simulink model "NPC_PI_SMO"  (R2021b)
settings: Solver=VariableStepAuto  StartTime=0.0  StopTime=3  RelTol=1e-3
values from neighbouring files (symbols this model uses):
  Cdc = 6000e-6    (= 0.006)    [Para_NPC_PI_SMO.m]
  Ki_a = 0.8    [Para_NPC_PI_SMO.m]
  Ki_b = 0    [Para_NPC_PI_SMO.m]
  Ki_c = 40    [Para_NPC_PI_SMO.m]
  Kp_a = 0.09    [Para_NPC_PI_SMO.m]
  Kp_b = 5e-3    (= 0.005)    [Para_NPC_PI_SMO.m]
  Kp_c = 10    [Para_NPC_PI_SMO.m]
  Lline = 2e-3    (= 0.002)    [Para_NPC_PI_SMO.m]
  rho = M + alpha*Cdc*0.3536    (= 10021.216)    [Para_NPC_PI_SMO.m]
  Tc = 1./fc    (= 0.0001)    [Para_NPC_PI_SMO.m]
  Tenable = 0.15    [Para_NPC_PI_SMO.m]
  Tint = 1e-6    (= 1e-06)    [Para_NPC_PI_SMO.m]
  Ts = 1./fs    (= 0.0001)    [Para_NPC_PI_SMO.m]
undefined symbols (not defined in the file or in its folder): DiscIntNeverNeededParam
libraries: spsNeutralLib x12, spsIGBTDiodeLib x12, spsSeriesRLCBranchLib x7, spsDiodeLib x6, slpidlib x4, spsBreakerLib x3, spsVoltageMeasurementLib x3, simulink x2, spsThreePhaseSeriesRLCBranchLib x2, spsabctodq0Lib x2, spsThreePhaseVIMeasurementLib x1, spsThreePhaseBreakerLib x1
settings Model: Creator=Taylor00225  LastModifiedBy=Taylor00225

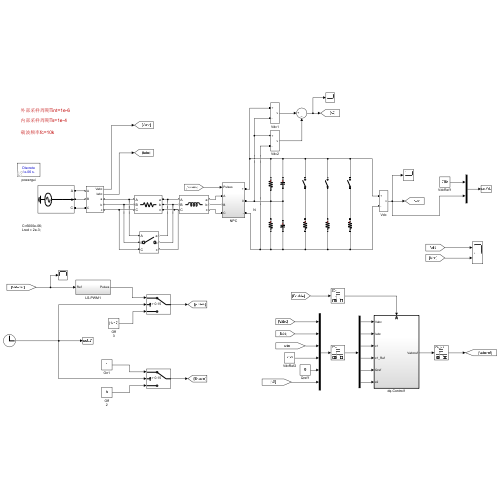
[thumbnail: Simulink's stored preview of the top-level diagram]
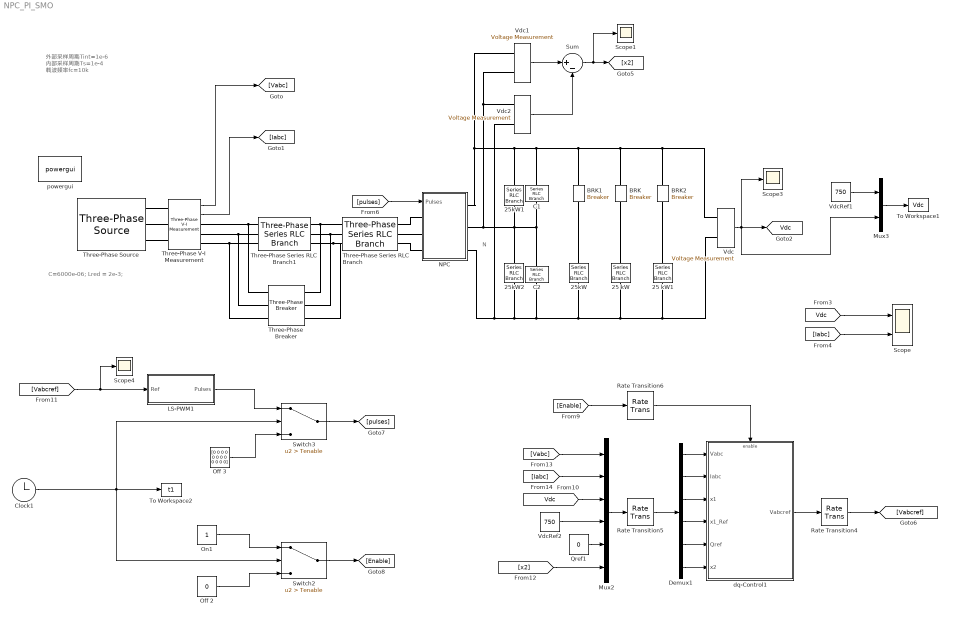
== system NPC_PI_SMO ==
  note: N
  note: 外部采样周期Tint=1e-6
      |
      | 内部采样周期Ts=1e-4
      |
      | 载波频率fc=10k
  note: C=6000e-06;
      | Lred = 2e-3;
  25 kW : spsSeriesRLCBranchLib/Series RLC Branch  LConnTagsString=__new0  RConnTagsString=__new0  BranchType=R  Resistance=360  Inductance=1.0  SetiL0=off  InitialCurrent=0  Capacitance=1.0  Setx0=off  InitialVoltage=0  Measurements=None
  25 kW1 : spsSeriesRLCBranchLib/Series RLC Branch  LConnTagsString=__new0  RConnTagsString=__new0  BranchType=R  Resistance=150  Inductance=1.0  SetiL0=off  InitialCurrent=0  Capacitance=1.0  Setx0=off  InitialVoltage=0  Measurements=None
  25kW : spsSeriesRLCBranchLib/Series RLC Branch  LConnTagsString=__new0  RConnTagsString=__new0  BranchType=R  Resistance=600  Inductance=1.0  SetiL0=off  InitialCurrent=0  Capacitance=1.0  Setx0=off  InitialVoltage=0  Measurements=None
  25kW1 : spsSeriesRLCBranchLib/Series RLC Branch  LConnTagsString=__new0  RConnTagsString=__new0  BranchType=R  Resistance=10e3  Inductance=1.0  SetiL0=off  InitialCurrent=0  Capacitance=1.0  Setx0=off  InitialVoltage=0  Measurements=None
  25kW2 : spsSeriesRLCBranchLib/Series RLC Branch  LConnTagsString=__new0  RConnTagsString=__new0  BranchType=R  Resistance=10e3  Inductance=1.0  SetiL0=off  InitialCurrent=0  Capacitance=1.0  Setx0=off  InitialVoltage=0  Measurements=None
  BRK : spsBreakerLib/Breaker  InitialState=0  SwitchingTimes=[1.2]  External=off  BreakerResistance=0.0001  SnubberResistance=inf  SnubberCapacitance=0  Measurements=None  MoreParameters=off  NoBreakLoop=off
      settings: SourceProductBaseCode=PS
  BRK1 : spsBreakerLib/Breaker  InitialState=0  SwitchingTimes=[0.7]  External=off  BreakerResistance=0.0001  SnubberResistance=inf  SnubberCapacitance=0  Measurements=None  MoreParameters=off  NoBreakLoop=off
      settings: SourceProductBaseCode=PS
  BRK2 : spsBreakerLib/Breaker  InitialState=0  SwitchingTimes=[1.9]  External=off  BreakerResistance=0.0001  SnubberResistance=inf  SnubberCapacitance=0  Measurements=None  MoreParameters=off  NoBreakLoop=off
      settings: SourceProductBaseCode=PS
  C1 : spsSeriesRLCBranchLib/Series RLC Branch  LConnTagsString=__new0  RConnTagsString=__new0  BranchType=C  Resistance=1.0  Inductance=1.0  SetiL0=off  InitialCurrent=0  Capacitance=6000e-06  Setx0=off  InitialVoltage=0  Measurements=None
  C2 : spsSeriesRLCBranchLib/Series RLC Branch  LConnTagsString=__new0  RConnTagsString=__new0  BranchType=C  Resistance=1.0  Inductance=1.0  SetiL0=off  InitialCurrent=0  Capacitance=6000e-06  Setx0=off  InitialVoltage=0  Measurements=None
  Clock1 : Clock
  Demux1 : Demux  Outputs=6
  LS-PWM1 : Subsystem
  Mux2 : Mux  Inputs=6
  Mux3 : Mux  Inputs=2
  NPC : Subsystem
  Off 2 : Constant  Value=0  SampleTime=Tint
  Off 3 : Constant  Value=[0 0 0 0 0 0 0 0 0 0 0 0]  SampleTime=Tint
  On1 : Constant  SampleTime=Tint
  Qref1 : Constant  Value=0  SampleTime=Tint
  Rate Transition4 : RateTransition  Deterministic=off  InitialCondition=[0 0 0]  OutPortSampleTime=Tint
  Rate Transition5 : RateTransition  OutPortSampleTime=Ts
  Rate Transition6 : RateTransition  OutPortSampleTime=Ts
  Scope : Scope  NumInputPorts=2
  Scope1 : Scope
  Scope3 : Scope
  Scope4 : Scope
  Sum : Sum  Inputs=|+-
  Switch2 : Switch  Criteria=u2 > Threshold  Threshold=Tenable
  Switch3 : Switch  Criteria=u2 > Threshold  Threshold=Tenable
  Three-Phase Series RLC Branch : spsThreePhaseSeriesRLCBranchLib/Three-Phase Series RLC Branch  LConnTagsString=A|B|C  RConnTagsString=A|B|C  BranchType=L  Resistance=1  Inductance=Lline  Capacitance=1e-6  Measurements=None
  Three-Phase Series RLC Branch1 : spsThreePhaseSeriesRLCBranchLib/Three-Phase Series RLC Branch  LConnTagsString=A|B|C  RConnTagsString=A|B|C  BranchType=R  Resistance=5  Inductance=2e-3  Capacitance=1e-6  Measurements=None
  Three-Phase V-I Measurement : spsThreePhaseVIMeasurementLib/Three-Phase V-I Measurement  VoltageMeasurement=phase-to-ground  SetLabelV=off  LabelV=Vabc  Vpu=off  VpuLL=off  CurrentMeasurement=yes  SetLabelI=off  LabelI=Iabc  Ipu=off  Pbase=100e6  Vbase=500e3  OutputType=Complex  PhasorSimulation=off  PSBequivalent=0
  Three-Phase Breaker : spsThreePhaseBreakerLib/Three-Phase Breaker  InitialState=open  SwitchA=on  SwitchB=on  SwitchC=on  SwitchTimes=[0.15]  External=off  BreakerResistance=0.00001  SnubberResistance=inf  SnubberCapacitance=0  Measurements=None
  Three-Phase Source : spsThreePhaseSourceLib/Three-Phase Source  InternalConnection=Yg  VoltagePhases=off  Voltage=400  PhaseAngle=0  Voltage_phases=[25e3 25e3 25e3]/sqrt(3)  PhaseAngles_phases=[0 -120 +120]  Frequency=50  NonIdealSource=on  SpecifyImpedance=off  Resistance=0  Inductance=0  ShortCircuitLevel=100e6  BaseVoltage=400  XRratio=7  BusType=swing  Pref=0  Qref=0  Prefabc=[10e3, 10e3, 10e3]  Qrefabc=[0, 0, 0]  Qmin=-inf  Qmax=inf
  To Workspace1 : ToWorkspace  VariableName=Vdc  SampleTime=-1
  To Workspace2 : ToWorkspace  VariableName=t1  SampleTime=-1
  Vdc : spsVoltageMeasurementLib/Voltage Measurement  PhasorSimulation=off  OutputType=Complex  PSBequivalent=0
  Vdc1 : spsVoltageMeasurementLib/Voltage Measurement  PhasorSimulation=off  OutputType=Complex  PSBequivalent=0
  Vdc2 : spsVoltageMeasurementLib/Voltage Measurement  PhasorSimulation=off  OutputType=Complex  PSBequivalent=0
  VdcRef1 : Constant  Value=750  SampleTime=Tint
  VdcRef2 : Constant  Value=750  SampleTime=Tint
  dq-Control1 : Subsystem  TreatAsAtomicUnit=on
  powergui : spspowerguiLib/powergui  Priority=1  SimulationMode=Discrete  SampleTime=Tint  frequency=60  Iterations=50  frequencyindice=0  Pbase=100e6  ErrMax=1e-4  UnitsV=kV  UnitsW=MW  buscounter=0  FunctionMessages=off  echomessages=off  EnableUseOfTLC=off  CurrentSourceSwitches=off  DisableSnubberDevices=off  DisableRonSwitches=off  DisableVfSwitches=off  DisplayEquations=off  AutomaticDiscreteSolvers=off  SolverType=Tustin  Interpol=off  ExternalGateDelay=off  methode=off  Ts=0  x0status=blocks  SPID=off  SwTol=0  HookPort=off  NonlinearTolerance=1e-4  nMaxIteration=100  ContinueOnMaxIteration=off  RestoreLinks=warning  ResistiveCurrentMeasurement=off  Frange=[0:2:500]  Ylog=off  Xlog=on  ShowGrid=off  save=off  variable=ZData  structure=ia  ZoomFFT=off  StartTime=1.9  cycles=5  DisplayStyle=1  fundamental=50  FreqAxis=on  MaxFrequency=2000  frequencyindicesteady=1  RmsSteady=1  display=off
  tag scope: Vdc=global
  wires:
  On1/1 -> Switch2/1
  Rate Transition4/1 -> [Vabcref]
  Off 2/1 -> Switch2/3
  Qref1/1 -> Mux2/5
  Switch3/1 -> [pulses]
  Rate Transition6/1 -> dq-Control1/Enable
  Demux1/6 -> dq-Control1/6(x2)
  Switch2/1 -> [Enable]
  [Enable] -> Rate Transition6/1
  Off 3/1 -> Switch3/3
  LS-PWM1/1(Pulses) -> Switch3/1
  [Vabc] -> Mux2/1
  [Vabcref] -> LS-PWM1/1(Ref), Scope4/1
  Demux1/1 -> dq-Control1/1(Vabc)
  Clock1/1 -> Switch2/2, Switch3/2, To Workspace2/1
  VdcRef2/1 -> Mux2/4
  [Vdc] -> Mux2/3
  Demux1/4 -> dq-Control1/4(x1_Ref)
  dq-Control1/1(Vabcref) -> Rate Transition4/1
  [Iabc] -> Mux2/2
  Mux2/1 -> Rate Transition5/1
  Demux1/2 -> dq-Control1/2(Iabc)
  Demux1/5 -> dq-Control1/5(Qref)
  Rate Transition5/1 -> Demux1/1
  Demux1/3 -> dq-Control1/3(x1)
  [x2] -> Mux2/6
  Sum/1 -> Scope1/1, [x2]
  Vdc2/1 -> Sum/2
  [Iabc] -> Scope/2
  VdcRef1/1 -> Mux3/1
  Three-Phase V-I Measurement/1 -> [Vabc]
  [pulses] -> NPC/1(Pulses)
  Vdc/1 -> Scope3/1, [Vdc], Mux3/2
  Three-Phase V-I Measurement/2 -> [Iabc]
  Vdc1/1 -> Sum/1
  Mux3/1 -> To Workspace1/1
  [Vdc] -> Scope/1
  connections:
  NPC/RConn3 -- Vdc2/LConn2 -- 25 kW/RConn1 -- Vdc/LConn2 -- 25 kW1/RConn1 -- 25kW/RConn1 -- C2/RConn1 -- 25kW2/RConn1
  Three-Phase Breaker/LConn2 -- Three-Phase V-I Measurement/RConn2 -- Three-Phase Series RLC Branch1/LConn2
  Three-Phase Breaker/RConn1 -- Three-Phase Series RLC Branch/LConn1 -- Three-Phase Series RLC Branch1/RConn1
  Three-Phase Breaker/LConn1 -- Three-Phase Series RLC Branch1/LConn1 -- Three-Phase V-I Measurement/RConn1
  Three-Phase Breaker/RConn3 -- Three-Phase Series RLC Branch/LConn3 -- Three-Phase Series RLC Branch1/RConn3
  Three-Phase Breaker/RConn2 -- Three-Phase Series RLC Branch1/RConn2 -- Three-Phase Series RLC Branch/LConn2
  Vdc1/LConn2 -- C1/RConn1 -- C2/LConn1 -- 25kW2/LConn1 -- 25kW1/RConn1 -- NPC/RConn2 -- Vdc2/LConn1
  Three-Phase Breaker/LConn3 -- Three-Phase Series RLC Branch1/LConn3 -- Three-Phase V-I Measurement/RConn3
  BRK/RConn1 -- BRK2/RConn1 -- Vdc/LConn1 -- C1/LConn1 -- 25kW1/LConn1 -- NPC/RConn1 -- Vdc1/LConn1 -- BRK1/RConn1
  BRK1/LConn1 -- 25kW/LConn1
  25 kW1/LConn1 -- BRK2/LConn1
  NPC/LConn1 -- Three-Phase Series RLC Branch/RConn1
  Three-Phase Source/RConn3 -- Three-Phase V-I Measurement/LConn3
  Three-Phase Source/RConn2 -- Three-Phase V-I Measurement/LConn2
  Three-Phase Source/RConn1 -- Three-Phase V-I Measurement/LConn1
  25 kW/LConn1 -- BRK/LConn1
  NPC/LConn2 -- Three-Phase Series RLC Branch/RConn2
  NPC/LConn3 -- Three-Phase Series RLC Branch/RConn3

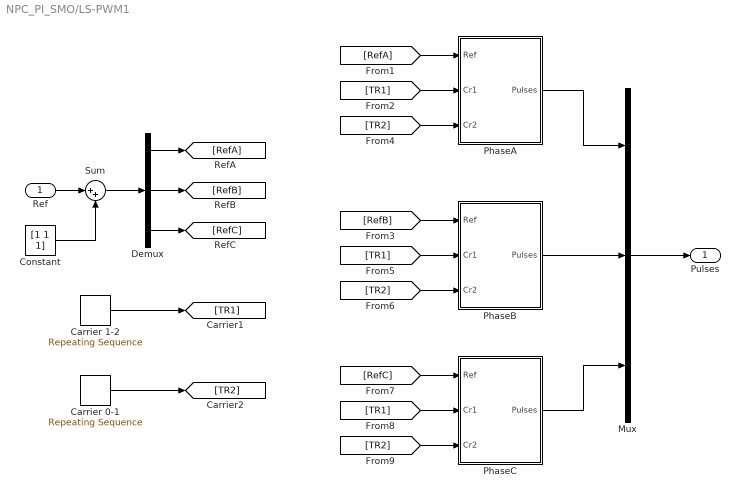
== system NPC_PI_SMO/LS-PWM1 ==
  Ref : Inport
  Carrier 0-1 : simulink/Sources/Repeating Sequence  rep_seq_t=[0 Tc/2 Tc]  rep_seq_y=[0 1 0]
  Carrier 1-2 : simulink/Sources/Repeating Sequence  rep_seq_t=[0 Tc/2 Tc]  rep_seq_y=[1 2 1]
  Constant : Constant  Value=[1 1 1]
  Demux : Demux  Outputs=3
  Mux : Mux  Inputs=3
  PhaseA : Subsystem
  PhaseB : Subsystem
  PhaseC : Subsystem
  Sum : Sum  Inputs=|++
  Pulses : Outport
  wires:
  Mux/1 -> Pulses/1
  PhaseC/1(Pulses) -> Mux/3
  PhaseA/1(Pulses) -> Mux/1
  PhaseB/1(Pulses) -> Mux/2
  [TR2] -> PhaseC/3(Cr2)
  [TR1] -> PhaseC/2(Cr1)
  [RefC] -> PhaseC/1(Ref)
  [TR2] -> PhaseB/3(Cr2)
  [TR1] -> PhaseB/2(Cr1)
  [RefB] -> PhaseB/1(Ref)
  [TR2] -> PhaseA/3(Cr2)
  [TR1] -> PhaseA/2(Cr1)
  [RefA] -> PhaseA/1(Ref)
  Constant/1 -> Sum/2
  Ref/1 -> Sum/1
  Sum/1 -> Demux/1
  Carrier 0-1/1 -> [TR2]
  Carrier 1-2/1 -> [TR1]
  Demux/3 -> [RefC]
  Demux/2 -> [RefB]
  Demux/1 -> [RefA]

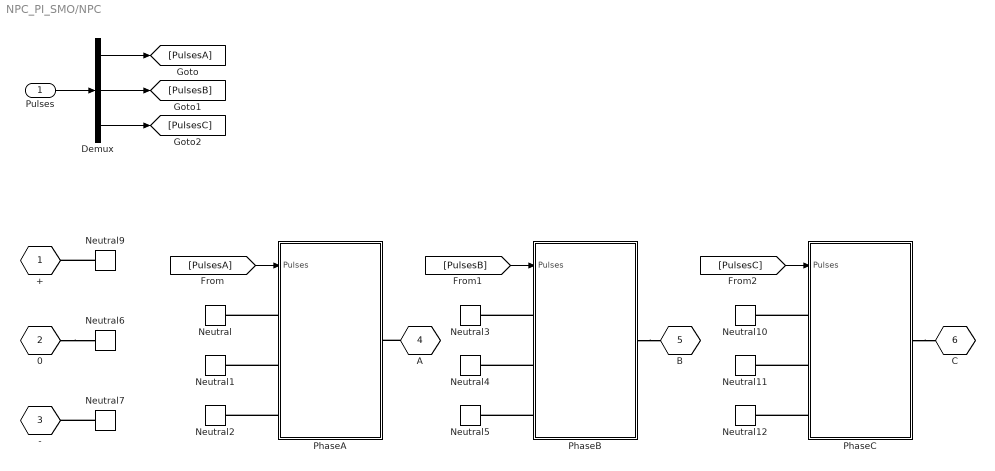
== system NPC_PI_SMO/NPC ==
  Pulses : Inport
  Demux : Demux  Outputs=3
  Neutral{,3,9..10} (4 alike) : spsNeutralLib/Neutral  LConnTagsString=a  NodeNumber=1
      settings: AttributesFormatString=node %<NodeNumber>  SourceProductBaseCode=PS
  Neutral{1,4,6,11} (4 alike) : spsNeutralLib/Neutral  LConnTagsString=a  NodeNumber=2
      settings: AttributesFormatString=node %<NodeNumber>  SourceProductBaseCode=PS
  Neutral{2,5,7,12} (4 alike) : spsNeutralLib/Neutral  LConnTagsString=a  NodeNumber=3
      settings: AttributesFormatString=node %<NodeNumber>  SourceProductBaseCode=PS
  PhaseA : Subsystem
  PhaseB : Subsystem
  PhaseC : Subsystem
  + : PMIOPort  Tag=PMCPort  Side=Right
  0 : PMIOPort  Tag=PMCPort  Port=2  Side=Right
  - : PMIOPort  Tag=PMCPort  Port=3  Side=Right
  A : PMIOPort  Tag=PMCPort  Port=4  Side=Left
  B : PMIOPort  Tag=PMCPort  Port=5  Side=Left
  C : PMIOPort  Tag=PMCPort  Port=6  Side=Left
  wires:
  Pulses/1 -> Demux/1
  Demux/1 -> [PulsesA]
  Demux/2 -> [PulsesB]
  Demux/3 -> [PulsesC]
  [PulsesA] -> PhaseA/1(Pulses)
  [PulsesB] -> PhaseB/1(Pulses)
  [PulsesC] -> PhaseC/1(Pulses)
  connections:
  PhaseA/LConn1 -- Neutral/LConn1
  PhaseA/LConn2 -- Neutral1/LConn1
  PhaseA/LConn3 -- Neutral2/LConn1
  PhaseB/LConn3 -- Neutral5/LConn1
  PhaseB/LConn1 -- Neutral3/LConn1
  PhaseB/LConn2 -- Neutral4/LConn1
  PhaseC/LConn2 -- Neutral11/LConn1
  PhaseC/LConn1 -- Neutral10/LConn1
  PhaseC/LConn3 -- Neutral12/LConn1
  Neutral9/LConn1 -- +/RConn1
  Neutral7/LConn1 -- -/RConn1
  0/RConn1 -- Neutral6/LConn1
  A/RConn1 -- PhaseA/RConn1
  PhaseB/RConn1 -- B/RConn1
  PhaseC/RConn1 -- C/RConn1

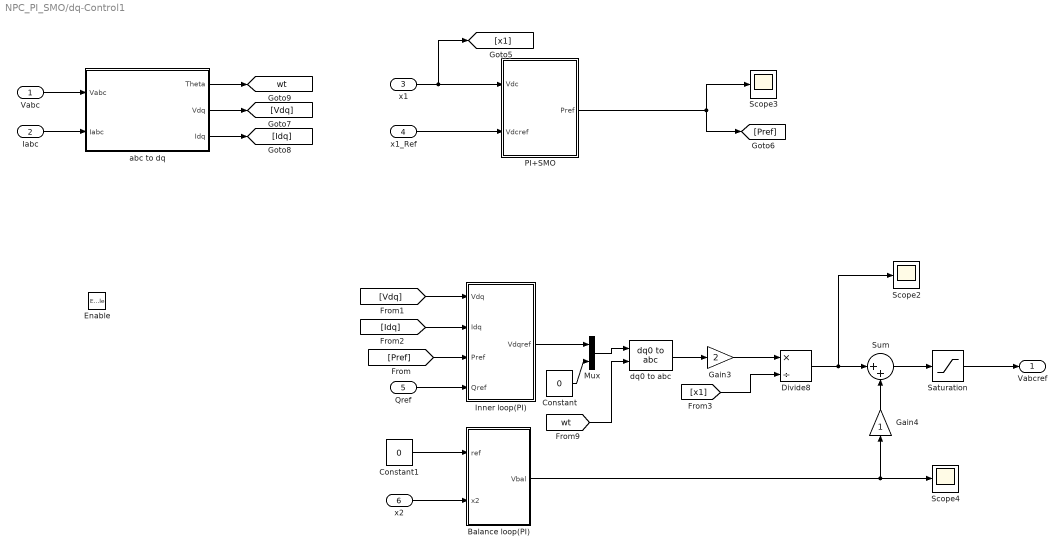
== system NPC_PI_SMO/dq-Control1 ==
  Vabc : Inport  PortDimensions=3
  Iabc : Inport  Port=2  PortDimensions=3
  x1 : Inport  Port=3  PortDimensions=1
  x1_Ref : Inport  Port=4  PortDimensions=1
  Qref : Inport  Port=5  PortDimensions=1
  x2 : Inport  Port=6  PortDimensions=1
  Enable : EnablePort
  Balance loop(PI) : Subsystem
  Constant : Constant  Value=0
  Constant1 : Constant  Value=0
  Divide8 : Product  Inputs=*/
  Gain3 : Gain  Gain=2
  Gain4 : Gain
  Inner loop(PI) : Subsystem
  Mux : Mux  Inputs=[2, 1]
  PI+SMO : Subsystem
  Saturation : Saturate  UpperLimit=1  LowerLimit=-1
  Scope2 : Scope
  Scope3 : Scope
  Scope4 : Scope
  Sum : Sum  Inputs=|++
  abc to dq : Subsystem  TreatAsAtomicUnit=on
  dq0 to abc : spsdq0toabcLib/dq0 to abc  Alignment=Aligned with phase A axis
  Vabcref : Outport  InitialOutput=[0 0 0]
  tag scope: wt=global
  wires:
  x1_Ref/1 -> PI+SMO/2(Vdcref)
  x1/1 -> [x1], PI+SMO/1(Vdc)
  Qref/1 -> Inner loop(PI)/4(Qref)
  [Pref] -> Inner loop(PI)/3(Pref)
  x2/1 -> Balance loop(PI)/2(x2)
  Balance loop(PI)/1(Vbal) -> Scope4/1, Gain4/1
  abc to dq/1(Theta) -> [wt]
  abc to dq/3(Idq) -> [Idq]
  Vabc/1 -> abc to dq/1(Vabc)
  Iabc/1 -> abc to dq/2(Iabc)
  [Vdq] -> Inner loop(PI)/1(Vdq)
  [Idq] -> Inner loop(PI)/2(Idq)
  [wt] -> dq0 to abc/2
  Gain3/1 -> Divide8/1
  Divide8/1 -> Scope2/1, Sum/1
  Sum/1 -> Saturation/1
  dq0 to abc/1 -> Gain3/1
  Saturation/1 -> Vabcref/1
  [x1] -> Divide8/2
  abc to dq/2(Vdq) -> [Vdq]
  Gain4/1 -> Sum/2
  Constant1/1 -> Balance loop(PI)/1(ref)
  PI+SMO/1(Pref) -> [Pref], Scope3/1
  Inner loop(PI)/1(Vdqref) -> Mux/1
  Constant/1 -> Mux/2
  Mux/1 -> dq0 to abc/1

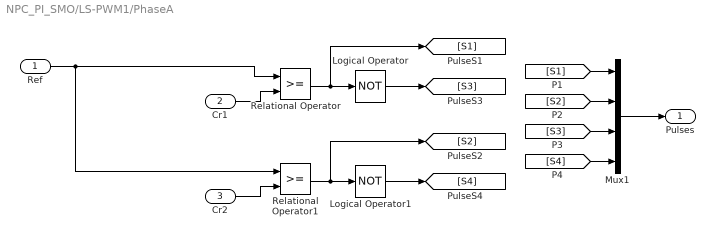
== system NPC_PI_SMO/LS-PWM1/PhaseA ==
  Ref : Inport
  Cr1 : Inport  Port=2
  Cr2 : Inport  Port=3
  Logical Operator : Logic  Operator=NOT  AllPortsSameDT=off  OutDataTypeStr=boolean
  Logical Operator1 : Logic  Operator=NOT  AllPortsSameDT=off  OutDataTypeStr=boolean
  Mux1 : Mux
  Relational Operator : RelationalOperator  OutDataTypeStr=boolean  RndMeth=Nearest
  Relational Operator1 : RelationalOperator  OutDataTypeStr=boolean  RndMeth=Nearest
  Pulses : Outport
  wires:
  Cr1/1 -> Relational Operator/2
  Relational Operator/1 -> Logical Operator/1, [S1]
  Logical Operator/1 -> [S3]
  Ref/1 -> Relational Operator1/1, Relational Operator/1
  Cr2/1 -> Relational Operator1/2
  Relational Operator1/1 -> Logical Operator1/1, [S2]
  Logical Operator1/1 -> [S4]
  Mux1/1 -> Pulses/1
  [S1] -> Mux1/1
  [S2] -> Mux1/2
  [S3] -> Mux1/3
  [S4] -> Mux1/4

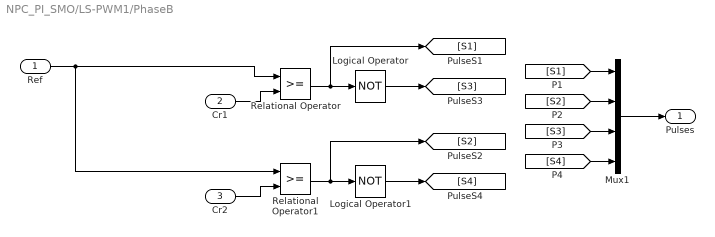
== system NPC_PI_SMO/LS-PWM1/PhaseB ==
  Ref : Inport
  Cr1 : Inport  Port=2
  Cr2 : Inport  Port=3
  Logical Operator : Logic  Operator=NOT  AllPortsSameDT=off  OutDataTypeStr=boolean
  Logical Operator1 : Logic  Operator=NOT  AllPortsSameDT=off  OutDataTypeStr=boolean
  Mux1 : Mux
  Relational Operator : RelationalOperator  OutDataTypeStr=boolean  RndMeth=Nearest
  Relational Operator1 : RelationalOperator  OutDataTypeStr=boolean  RndMeth=Nearest
  Pulses : Outport
  wires:
  [S4] -> Mux1/4
  [S3] -> Mux1/3
  [S2] -> Mux1/2
  [S1] -> Mux1/1
  Mux1/1 -> Pulses/1
  Logical Operator1/1 -> [S4]
  Relational Operator1/1 -> [S2], Logical Operator1/1
  Cr2/1 -> Relational Operator1/2
  Ref/1 -> Relational Operator/1, Relational Operator1/1
  Logical Operator/1 -> [S3]
  Relational Operator/1 -> [S1], Logical Operator/1
  Cr1/1 -> Relational Operator/2

== system NPC_PI_SMO/LS-PWM1/PhaseC ==
  Ref : Inport
  Cr1 : Inport  Port=2
  Cr2 : Inport  Port=3
  Logical Operator : Logic  Operator=NOT  AllPortsSameDT=off  OutDataTypeStr=boolean
  Logical Operator1 : Logic  Operator=NOT  AllPortsSameDT=off  OutDataTypeStr=boolean
  Mux1 : Mux
  Relational Operator : RelationalOperator  OutDataTypeStr=boolean  RndMeth=Nearest
  Relational Operator1 : RelationalOperator  OutDataTypeStr=boolean  RndMeth=Nearest
  Pulses : Outport
  wires:
  Cr1/1 -> Relational Operator/2
  Relational Operator/1 -> Logical Operator/1, [S1]
  Logical Operator/1 -> [S3]
  Ref/1 -> Relational Operator1/1, Relational Operator/1
  Cr2/1 -> Relational Operator1/2
  Relational Operator1/1 -> Logical Operator1/1, [S2]
  Logical Operator1/1 -> [S4]
  Mux1/1 -> Pulses/1
  [S1] -> Mux1/1
  [S2] -> Mux1/2
  [S3] -> Mux1/3
  [S4] -> Mux1/4

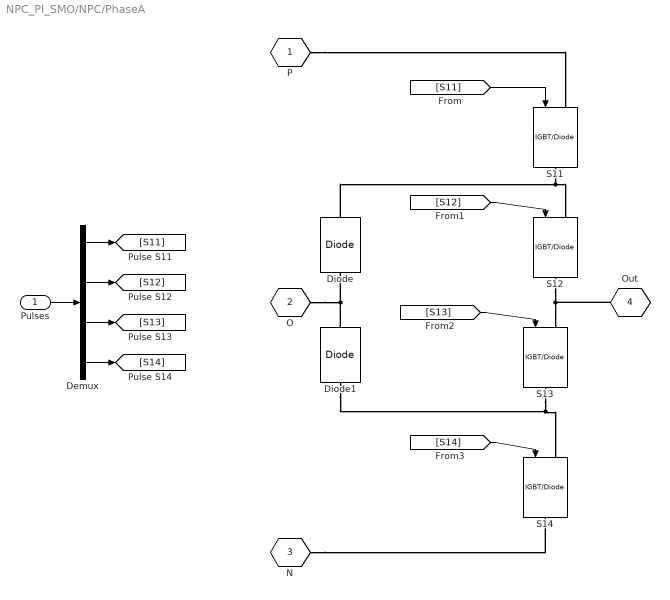
== system NPC_PI_SMO/NPC/PhaseA ==
  Pulses : Inport
  Demux : Demux
  Diode : spsDiodeLib/Diode  Ron=0.001  Lon=0  Vf=0.8  IC=0  UseSnubber=off  Rs=1e5  Cs=inf  Measurements=off
  Diode1 : spsDiodeLib/Diode  Ron=0.001  Lon=0  Vf=0.8  IC=0  UseSnubber=off  Rs=1e5  Cs=inf  Measurements=off
  S{11..14} (4 alike) : spsIGBTDiodeLib/IGBT//Diode  Ron=1e-3  Rs=1e5  Cs=inf  Measurements=off
  P : PMIOPort  Tag=PMCPort  Side=Left
  O : PMIOPort  Tag=PMCPort  Port=2  Side=Left
  N : PMIOPort  Tag=PMCPort  Port=3  Side=Left
  Out : PMIOPort  Tag=PMCPort  Port=4  Side=Right
  wires:
  Pulses/1 -> Demux/1
  Demux/1 -> [S11]
  Demux/3 -> [S13]
  Demux/2 -> [S12]
  Demux/4 -> [S14]
  [S11] -> S11/1
  [S12] -> S12/1
  [S13] -> S13/1
  [S14] -> S14/1
  connections:
  S11/RConn1 -- S12/LConn1 -- Diode/RConn1
  S13/RConn1 -- Diode1/LConn1 -- S14/LConn1
  Diode1/RConn1 -- O/RConn1 -- Diode/LConn1
  S12/RConn1 -- Out/RConn1 -- S13/LConn1
  P/RConn1 -- S11/LConn1
  N/RConn1 -- S14/RConn1

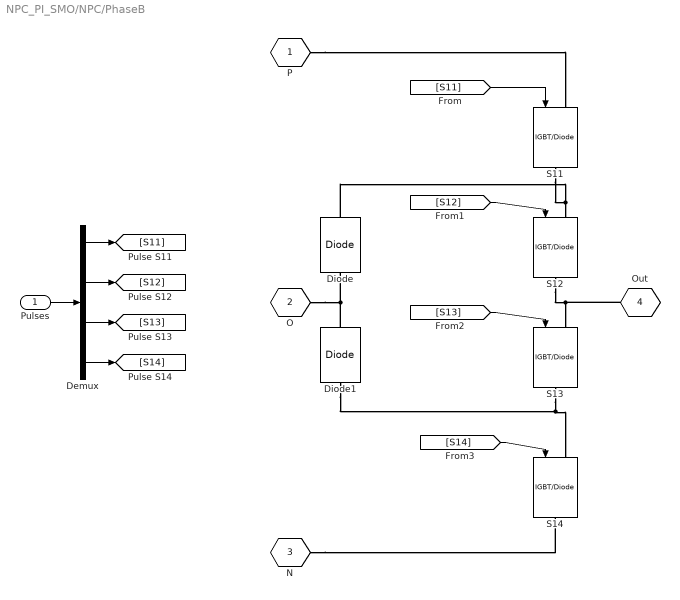
== system NPC_PI_SMO/NPC/PhaseB ==
  Pulses : Inport
  Demux : Demux
  Diode : spsDiodeLib/Diode  Ron=0.001  Lon=0  Vf=0.8  IC=0  UseSnubber=off  Rs=1e5  Cs=inf  Measurements=off
  Diode1 : spsDiodeLib/Diode  Ron=0.001  Lon=0  Vf=0.8  IC=0  UseSnubber=off  Rs=1e5  Cs=inf  Measurements=off
  S{11..14} (4 alike) : spsIGBTDiodeLib/IGBT//Diode  Ron=1e-3  Rs=1e5  Cs=inf  Measurements=off
  P : PMIOPort  Tag=PMCPort  Side=Left
  O : PMIOPort  Tag=PMCPort  Port=2  Side=Left
  N : PMIOPort  Tag=PMCPort  Port=3  Side=Left
  Out : PMIOPort  Tag=PMCPort  Port=4  Side=Right
  wires:
  [S14] -> S14/1
  [S13] -> S13/1
  [S12] -> S12/1
  [S11] -> S11/1
  Demux/4 -> [S14]
  Demux/2 -> [S12]
  Demux/3 -> [S13]
  Demux/1 -> [S11]
  Pulses/1 -> Demux/1
  connections:
  N/RConn1 -- S14/RConn1
  P/RConn1 -- S11/LConn1
  Out/RConn1 -- S13/LConn1 -- S12/RConn1
  O/RConn1 -- Diode1/RConn1 -- Diode/LConn1
  Diode1/LConn1 -- S13/RConn1 -- S14/LConn1
  S12/LConn1 -- S11/RConn1 -- Diode/RConn1

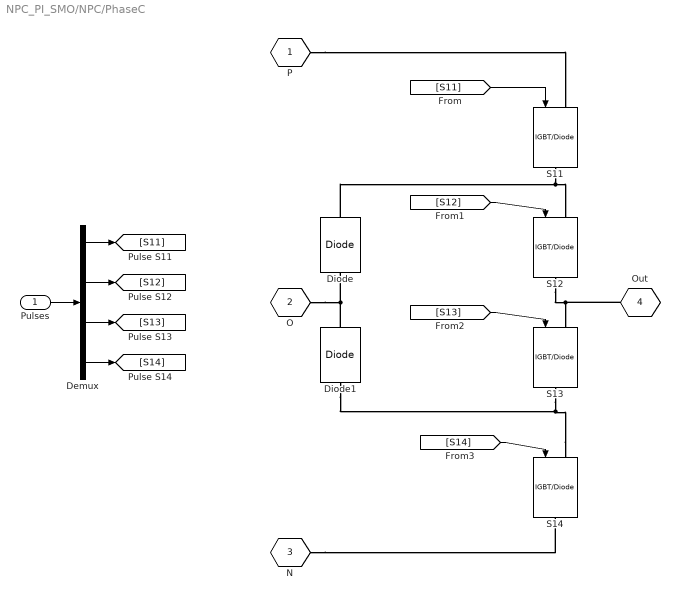
== system NPC_PI_SMO/NPC/PhaseC ==
  Pulses : Inport
  Demux : Demux
  Diode : spsDiodeLib/Diode  Ron=0.001  Lon=0  Vf=0.8  IC=0  UseSnubber=off  Rs=1e5  Cs=inf  Measurements=off
  Diode1 : spsDiodeLib/Diode  Ron=0.001  Lon=0  Vf=0.8  IC=0  UseSnubber=off  Rs=1e5  Cs=inf  Measurements=off
  S{11..14} (4 alike) : spsIGBTDiodeLib/IGBT//Diode  Ron=1e-3  Rs=1e5  Cs=inf  Measurements=off
  P : PMIOPort  Tag=PMCPort  Side=Left
  O : PMIOPort  Tag=PMCPort  Port=2  Side=Left
  N : PMIOPort  Tag=PMCPort  Port=3  Side=Left
  Out : PMIOPort  Tag=PMCPort  Port=4  Side=Right
  wires:
  Pulses/1 -> Demux/1
  Demux/1 -> [S11]
  Demux/3 -> [S13]
  Demux/2 -> [S12]
  Demux/4 -> [S14]
  [S11] -> S11/1
  [S12] -> S12/1
  [S13] -> S13/1
  [S14] -> S14/1
  connections:
  Diode/RConn1 -- S11/RConn1 -- S12/LConn1
  S14/LConn1 -- S13/RConn1 -- Diode1/LConn1
  Diode/LConn1 -- Diode1/RConn1 -- O/RConn1
  S12/RConn1 -- S13/LConn1 -- Out/RConn1
  P/RConn1 -- S11/LConn1
  N/RConn1 -- S14/RConn1

== system NPC_PI_SMO/dq-Control1/Balance loop(PI) ==
  ref : Inport
  x2 : Inport  Port=2
  PID Controller4 : slpidlib/PID Controller  Controller=PID  Form=Parallel  TimeDomain=Discrete-time  UseExternalTs=off  SampleTime=Ts  IntegratorMethod=Forward Euler  FilterMethod=Forward Euler  ControllerParametersSource=internal  P=Kp_b  I=Ki_b  D=0  UseFilter=on  N=0  TunerSelectOption=Transfer Function Based (PID Tuner App)  InitialConditionSource=internal  InitialConditionForIntegrator=0  InitialConditionForFilter=0  DifferentiatorICPrevScaledInput=0  ExternalReset=none  TrackingMode=off  Kt=1  LimitOutput=off  SatLimitsSource=internal  UpperSaturationLimit=inf  LowerSaturationLimit=-inf  LinearizeAsGain=on  AntiWindupMode=none  Kb=1  POutMin=[]  POutMax=[]  IOutMin=[]  IOutMax=[]  DOutMin=[]  DOutMax=[]  NOutMin=[]  NOutMax=[]  SumOutMin=[]  SumOutMax=[]  SaturationOutMin=[]  SaturationOutMax=[]  PParamMin=[]  PParamMax=[]  IParamMin=[]  IParamMax=[]  DParamMin=[]  DParamMax=[]  NParamMin=[]  NParamMax=[]  KbParamMin=[]  KbParamMax=[]  KtParamMin=[]  KtParamMax=[]  KbOutMin=[]  KbOutMax=[]  KtOutMin=[]  KtOutMax=[]  IntegratorOutMin=[]  IntegratorOutMax=[]  FilterOutMin=[]  FilterOutMax=[]  SumI1OutMin=[]  SumI1OutMax=[]  SumI2OutMin=[]  SumI2OutMax=[]  SumI3OutMin=[]  SumI3OutMax=[]  SumI4OutMin=[]  SumI4OutMax=[]  SumDOutMin=[]  SumDOutMax=[]  DifferentiatorOutMin=[]  DifferentiatorOutMax=[]  FilterDiffOutCoefMin=[]  FilterDiffOutCoefMax=[]  ReciprocalOutMin=[]  ReciprocalOutMax=[]  SumDenOutMin=[]  SumDenOutMax=[]  SumNumOutMin=[]  SumNumOutMax=[]  DivideOutMin=[]  DivideOutMax=[]  UdiffTsProdOutMin=[]  UdiffTsProdOutMax=[]  NTsProdOutMin=[]  NTsProdOutMax=[]  UintegralTsProdOutMin=[]  UintegralTsProdOutMax=[]  UngainTsProdOutMin=[]  UngainTsProdOutMax=[]  IntegratorContinuousStateAttributes=''  IntegratorStateMustResolveToSignalObject=off  IntegratorRTWStateStorageClass=Auto  FilterContinuousStateAttributes=''  FilterStateMustResolveToSignalObject=off  FilterRTWStateStorageClass=Auto  ParallelPVariant=InternalParameters  IdealPVariant=Disabled  IVariant=InternalParameters  DVariant=InternalParameters  IntegratorVariant=Discrete  SatVariant=Disabled  AWVariant=Passthrough  PCopyVariant=Disabled  TRVariant=Disabled  FdbkBlocksVariant=Forward  IdealPFdbkVariant=Disabled  SatFdbkVariant=Disabled  DerivativeFilterVariant=ForwardEulerFilter  NVariant=InternalParameters  NCopyVariant=Disabled  FilterICVariant=InternalICsFilter  IntegratorICVariant=InternalICs  ExternalResetVariant=Disabled  TRSumVariant=Passthrough  SumFdbkVariant=Disabled  SumVariant=Sum_PID  TsampFilterVariant=InternalTs  TsampNgainVariant=Passthrough  TsampIntegralVariant=Passthrough  ExternalSaturationOutDataTypeStr=Inherit: Same as second input
  Sum1 : Sum  Inputs=|+-
  Vbal : Outport
  wires:
  PID Controller4/1 -> Vbal/1
  ref/1 -> Sum1/1
  x2/1 -> Sum1/2
  Sum1/1 -> PID Controller4/1

== system NPC_PI_SMO/dq-Control1/Inner loop(PI) ==
  Vdq : Inport
  Idq : Inport  Port=2
  Pref : Inport  Port=3
  Qref : Inport  Port=4
  Demux : Demux  Outputs=2
  Demux1 : Demux  Outputs=2
  Idq Control : Subsystem
  Idqref Calculation : Subsystem
  Mux : Mux  Inputs=2
  Scope3 : Scope
  Vdqref : Outport  InitialOutput=[0 0 0]
  wires:
  Vdq/1 -> Idqref Calculation/1(Vdq)
  Qref/1 -> Idqref Calculation/3(Qref)
  Pref/1 -> Idqref Calculation/2(Pref)
  Idqref Calculation/1(IdqRef) -> [Idqref]
  [Idqref] -> Idq Control/1(Idqref), Demux1/1
  Idq/1 -> Demux/1, Idq Control/2(Idq)
  Idq Control/1(Vdqref) -> Vdqref/1
  Demux1/1 -> Mux/1
  Demux/1 -> Mux/2
  Mux/1 -> Scope3/1

== system NPC_PI_SMO/dq-Control1/PI+SMO ==
  Vdc : Inport
  Vdcref : Inport  Port=2
  Discrete PID Controller : slpidlib/PID Controller  Controller=PI  Form=Parallel  TimeDomain=Discrete-time  UseExternalTs=off  SampleTime=-1  IntegratorMethod=Forward Euler  FilterMethod=Forward Euler  ControllerParametersSource=internal  P=Kp_a  I=Ki_a  D=0  UseFilter=on  N=0  TunerSelectOption=Transfer Function Based (PID Tuner App)  InitialConditionSource=internal  InitialConditionForIntegrator=0  InitialConditionForFilter=0  DifferentiatorICPrevScaledInput=0  ExternalReset=none  TrackingMode=off  Kt=1  LimitOutput=off  SatLimitsSource=internal  UpperSaturationLimit=inf  LowerSaturationLimit=-inf  LinearizeAsGain=off  AntiWindupMode=none  Kb=1  POutMin=[]  POutMax=[]  IOutMin=[]  IOutMax=[]  DOutMin=[]  DOutMax=[]  NOutMin=[]  NOutMax=[]  SumOutMin=[]  SumOutMax=[]  SaturationOutMin=[]  SaturationOutMax=[]  PParamMin=[]  PParamMax=[]  IParamMin=[]  IParamMax=[]  DParamMin=[]  DParamMax=[]  NParamMin=[]  NParamMax=[]  KbParamMin=[]  KbParamMax=[]  KtParamMin=[]  KtParamMax=[]  KbOutMin=[]  KbOutMax=[]  KtOutMin=[]  KtOutMax=[]  IntegratorOutMin=[]  IntegratorOutMax=[]  FilterOutMin=[]  FilterOutMax=[]  SumI1OutMin=[]  SumI1OutMax=[]  SumI2OutMin=[]  SumI2OutMax=[]  SumI3OutMin=[]  SumI3OutMax=[]  SumI4OutMin=[]  SumI4OutMax=[]  SumDOutMin=[]  SumDOutMax=[]  DifferentiatorOutMin=[]  DifferentiatorOutMax=[]  FilterDiffOutCoefMin=[]  FilterDiffOutCoefMax=[]  ReciprocalOutMin=[]  ReciprocalOutMax=[]  SumDenOutMin=[]  SumDenOutMax=[]  SumNumOutMin=[]  SumNumOutMax=[]  DivideOutMin=[]  DivideOutMax=[]  UdiffTsProdOutMin=[]  UdiffTsProdOutMax=[]  NTsProdOutMin=[]  NTsProdOutMax=[]  UintegralTsProdOutMin=[]  UintegralTsProdOutMax=[]  UngainTsProdOutMin=[]  UngainTsProdOutMax=[]  IntegratorContinuousStateAttributes=''  IntegratorStateMustResolveToSignalObject=off  IntegratorRTWStateStorageClass=Auto  FilterContinuousStateAttributes=''  FilterStateMustResolveToSignalObject=off  FilterRTWStateStorageClass=Auto  ParallelPVariant=InternalParameters  IdealPVariant=Disabled  IVariant=InternalParameters  DVariant=Disabled  IntegratorVariant=Discrete  SatVariant=Disabled  AWVariant=Passthrough  PCopyVariant=Disabled  TRVariant=Disabled  FdbkBlocksVariant=Forward  IdealPFdbkVariant=Disabled  SatFdbkVariant=Disabled  DerivativeFilterVariant=Disabled  NVariant=Disabled  NCopyVariant=Disabled_SignalSpec  FilterICVariant=Disabled  IntegratorICVariant=InternalICs  ExternalResetVariant=Disabled  TRSumVariant=Passthrough  SumFdbkVariant=Disabled  SumVariant=Sum_PI  TsampFilterVariant=InternalTs  TsampNgainVariant=Passthrough  TsampIntegralVariant=Passthrough  ExternalSaturationOutDataTypeStr=Inherit: Same as second input
  Gain : Gain  Gain=0.5
  Gain2 : Gain  Gain=0.5
  Product : Product
  Product1 : Product
  SMO : Subsystem
  Sum : Sum  Inputs=|-+
  Sum1 : Sum  Inputs=|++
  Pref : Outport
  wires:
  Discrete PID Controller/1 -> Sum1/1, SMO/1(ud)
  [zref] -> Sum/2
  Gain2/1 -> [zref]
  Product1/1 -> Gain2/1
  Gain/1 -> [z]
  Product/1 -> Gain/1
  Vdcref/1 -> Product1/1, Product1/2
  Vdc/1 -> Product/1, Product/2
  Sum/1 -> Discrete PID Controller/1
  [z] -> SMO/2(y)
  Sum1/1 -> Pref/1
  [z] -> Sum/1
  SMO/1(disturb) -> Sum1/2

== system NPC_PI_SMO/dq-Control1/abc to dq ==
  Vabc : Inport
  Iabc : Inport  Port=2
  Demux : Demux  Outputs=[2, 1]
  Demux1 : Demux  Outputs=[2, 1]
  PLL (3ph) : spsPLL3phLib/PLL (3ph)  Fmin=45  Par_Init=[0, 50]  ParK=[180, 3200, 1]  TcD=1e-4  MaxRateChangeFreq=12  FilterCutOffFreq=25  Ts=Ts  AGC=on
  abc to dq0 : spsabctodq0Lib/abc to dq0  Alignment=Aligned with phase A axis
  abc to dq1 : spsabctodq0Lib/abc to dq0  Alignment=Aligned with phase A axis
  Theta : Outport
  Vdq : Outport  Port=2
  Idq : Outport  Port=3
  wires:
  Vabc/1 -> abc to dq0/1, PLL (3ph)/1
  [Theta] -> Theta/1
  PLL (3ph)/2 -> abc to dq0/2, [Theta]
  Iabc/1 -> abc to dq1/1
  [Theta] -> abc to dq1/2
  abc to dq0/1 -> Demux/1
  Demux/1 -> Vdq/1
  abc to dq1/1 -> Demux1/1
  Demux1/1 -> Idq/1

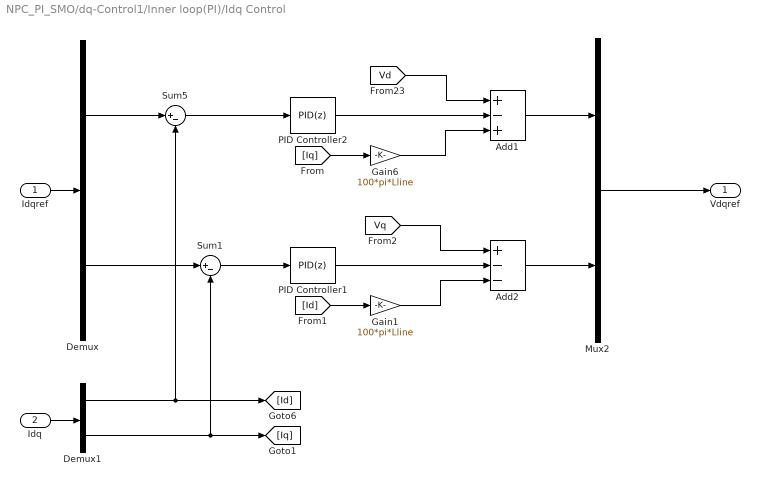
== system NPC_PI_SMO/dq-Control1/Inner loop(PI)/Idq Control ==
  Idqref : Inport
  Idq : Inport  Port=2
  Add1 : Sum  Inputs=+-+
  Add2 : Sum  Inputs=+--
  Demux : Demux  Outputs=2
  Demux1 : Demux  Outputs=2
  Gain1 : Gain  Gain=100*pi*Lline
  Gain6 : Gain  Gain=100*pi*Lline
  Mux2 : Mux  Inputs=2
  PID Controller1 : slpidlib/PID Controller  Controller=PID  Form=Parallel  TimeDomain=Discrete-time  UseExternalTs=off  SampleTime=Ts  IntegratorMethod=Forward Euler  FilterMethod=Forward Euler  ControllerParametersSource=internal  P=Kp_c  I=Ki_c  D=0  UseFilter=on  N=0  TunerSelectOption=Transfer Function Based (PID Tuner App)  InitialConditionSource=internal  InitialConditionForIntegrator=0  InitialConditionForFilter=0  DifferentiatorICPrevScaledInput=0  ExternalReset=none  TrackingMode=off  Kt=1  LimitOutput=off  SatLimitsSource=internal  UpperSaturationLimit=inf  LowerSaturationLimit=-inf  LinearizeAsGain=on  AntiWindupMode=none  Kb=1  POutMin=[]  POutMax=[]  IOutMin=[]  IOutMax=[]  DOutMin=[]  DOutMax=[]  NOutMin=[]  NOutMax=[]  SumOutMin=[]  SumOutMax=[]  SaturationOutMin=[]  SaturationOutMax=[]  PParamMin=[]  PParamMax=[]  IParamMin=[]  IParamMax=[]  DParamMin=[]  DParamMax=[]  NParamMin=[]  NParamMax=[]  KbParamMin=[]  KbParamMax=[]  KtParamMin=[]  KtParamMax=[]  KbOutMin=[]  KbOutMax=[]  KtOutMin=[]  KtOutMax=[]  IntegratorOutMin=[]  IntegratorOutMax=[]  FilterOutMin=[]  FilterOutMax=[]  SumI1OutMin=[]  SumI1OutMax=[]  SumI2OutMin=[]  SumI2OutMax=[]  SumI3OutMin=[]  SumI3OutMax=[]  SumI4OutMin=[]  SumI4OutMax=[]  SumDOutMin=[]  SumDOutMax=[]  DifferentiatorOutMin=[]  DifferentiatorOutMax=[]  FilterDiffOutCoefMin=[]  FilterDiffOutCoefMax=[]  ReciprocalOutMin=[]  ReciprocalOutMax=[]  SumDenOutMin=[]  SumDenOutMax=[]  SumNumOutMin=[]  SumNumOutMax=[]  DivideOutMin=[]  DivideOutMax=[]  UdiffTsProdOutMin=[]  UdiffTsProdOutMax=[]  NTsProdOutMin=[]  NTsProdOutMax=[]  UintegralTsProdOutMin=[]  UintegralTsProdOutMax=[]  UngainTsProdOutMin=[]  UngainTsProdOutMax=[]  IntegratorContinuousStateAttributes=''  IntegratorStateMustResolveToSignalObject=off  IntegratorRTWStateStorageClass=Auto  FilterContinuousStateAttributes=''  FilterStateMustResolveToSignalObject=off  FilterRTWStateStorageClass=Auto  ParallelPVariant=InternalParameters  IdealPVariant=Disabled  IVariant=InternalParameters  DVariant=InternalParameters  IntegratorVariant=Discrete  SatVariant=Disabled  AWVariant=Passthrough  PCopyVariant=Disabled  TRVariant=Disabled  FdbkBlocksVariant=Forward  IdealPFdbkVariant=Disabled  SatFdbkVariant=Disabled  DerivativeFilterVariant=ForwardEulerFilter  NVariant=InternalParameters  NCopyVariant=Disabled  FilterICVariant=InternalICsFilter  IntegratorICVariant=InternalICs  ExternalResetVariant=Disabled  TRSumVariant=Passthrough  SumFdbkVariant=Disabled  SumVariant=Sum_PID  TsampFilterVariant=InternalTs  TsampNgainVariant=Passthrough  TsampIntegralVariant=Passthrough  ExternalSaturationOutDataTypeStr=Inherit: Same as second input
  PID Controller2 : slpidlib/PID Controller  Controller=PID  Form=Parallel  TimeDomain=Discrete-time  UseExternalTs=off  SampleTime=Ts  IntegratorMethod=Forward Euler  FilterMethod=Forward Euler  ControllerParametersSource=internal  P=Kp_c  I=Ki_c  D=0  UseFilter=on  N=0  TunerSelectOption=Transfer Function Based (PID Tuner App)  InitialConditionSource=internal  InitialConditionForIntegrator=0  InitialConditionForFilter=0  DifferentiatorICPrevScaledInput=0  ExternalReset=none  TrackingMode=off  Kt=1  LimitOutput=off  SatLimitsSource=internal  UpperSaturationLimit=inf  LowerSaturationLimit=-inf  LinearizeAsGain=on  AntiWindupMode=none  Kb=1  POutMin=[]  POutMax=[]  IOutMin=[]  IOutMax=[]  DOutMin=[]  DOutMax=[]  NOutMin=[]  NOutMax=[]  SumOutMin=[]  SumOutMax=[]  SaturationOutMin=[]  SaturationOutMax=[]  PParamMin=[]  PParamMax=[]  IParamMin=[]  IParamMax=[]  DParamMin=[]  DParamMax=[]  NParamMin=[]  NParamMax=[]  KbParamMin=[]  KbParamMax=[]  KtParamMin=[]  KtParamMax=[]  KbOutMin=[]  KbOutMax=[]  KtOutMin=[]  KtOutMax=[]  IntegratorOutMin=[]  IntegratorOutMax=[]  FilterOutMin=[]  FilterOutMax=[]  SumI1OutMin=[]  SumI1OutMax=[]  SumI2OutMin=[]  SumI2OutMax=[]  SumI3OutMin=[]  SumI3OutMax=[]  SumI4OutMin=[]  SumI4OutMax=[]  SumDOutMin=[]  SumDOutMax=[]  DifferentiatorOutMin=[]  DifferentiatorOutMax=[]  FilterDiffOutCoefMin=[]  FilterDiffOutCoefMax=[]  ReciprocalOutMin=[]  ReciprocalOutMax=[]  SumDenOutMin=[]  SumDenOutMax=[]  SumNumOutMin=[]  SumNumOutMax=[]  DivideOutMin=[]  DivideOutMax=[]  UdiffTsProdOutMin=[]  UdiffTsProdOutMax=[]  NTsProdOutMin=[]  NTsProdOutMax=[]  UintegralTsProdOutMin=[]  UintegralTsProdOutMax=[]  UngainTsProdOutMin=[]  UngainTsProdOutMax=[]  IntegratorContinuousStateAttributes=''  IntegratorStateMustResolveToSignalObject=off  IntegratorRTWStateStorageClass=Auto  FilterContinuousStateAttributes=''  FilterStateMustResolveToSignalObject=off  FilterRTWStateStorageClass=Auto  ParallelPVariant=InternalParameters  IdealPVariant=Disabled  IVariant=InternalParameters  DVariant=InternalParameters  IntegratorVariant=Discrete  SatVariant=Disabled  AWVariant=Passthrough  PCopyVariant=Disabled  TRVariant=Disabled  FdbkBlocksVariant=Forward  IdealPFdbkVariant=Disabled  SatFdbkVariant=Disabled  DerivativeFilterVariant=ForwardEulerFilter  NVariant=InternalParameters  NCopyVariant=Disabled  FilterICVariant=InternalICsFilter  IntegratorICVariant=InternalICs  ExternalResetVariant=Disabled  TRSumVariant=Passthrough  SumFdbkVariant=Disabled  SumVariant=Sum_PID  TsampFilterVariant=InternalTs  TsampNgainVariant=Passthrough  TsampIntegralVariant=Passthrough  ExternalSaturationOutDataTypeStr=Inherit: Same as second input
  Sum1 : Sum  Inputs=|+-
  Sum5 : Sum  Inputs=|+-
  Vdqref : Outport
  wires:
  Idqref/1 -> Demux/1
  Idq/1 -> Demux1/1
  Demux/1 -> Sum5/1
  Demux1/1 -> [Id], Sum5/2
  Demux/2 -> Sum1/1
  Demux1/2 -> [Iq], Sum1/2
  Sum5/1 -> PID Controller2/1
  Sum1/1 -> PID Controller1/1
  [Iq] -> Gain6/1
  [Id] -> Gain1/1
  PID Controller2/1 -> Add1/2
  [Vd] -> Add1/1
  Gain6/1 -> Add1/3
  PID Controller1/1 -> Add2/2
  [Vq] -> Add2/1
  Gain1/1 -> Add2/3
  Add1/1 -> Mux2/1
  Add2/1 -> Mux2/2
  Mux2/1 -> Vdqref/1

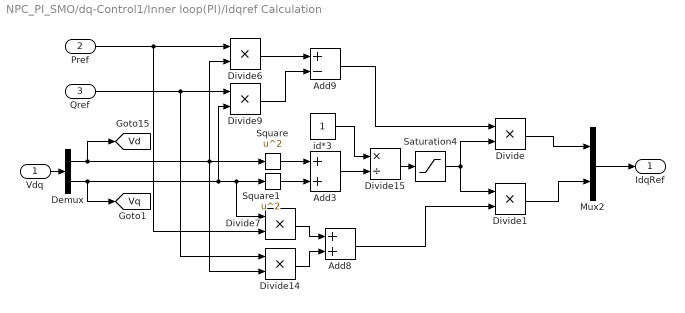
== system NPC_PI_SMO/dq-Control1/Inner loop(PI)/Idqref Calculation ==
  Vdq : Inport
  Pref : Inport  Port=2
  Qref : Inport  Port=3
  Add3 : Sum
  Add8 : Sum
  Add9 : Sum  Inputs=+-
  Demux : Demux  Outputs=2
  Divide{,1,6..7,9,14} (6 alike) : Product  Inputs=**
  Divide15 : Product  Inputs=*/
  Mux2 : Mux  Inputs=2
  Saturation4 : Saturate  UpperLimit=10e6  LowerLimit=1e-7
  Square : Math  Operator=square  SignedPower=on  RndMeth=Zero  SaturateOnIntegerOverflow=on
  Square1 : Math  Operator=square  SignedPower=on  RndMeth=Zero  SaturateOnIntegerOverflow=on
  id*3 : Constant
  IdqRef : Outport
  tag scope: Vd=global, Vq=global
  wires:
  Demux/2 -> [Vq], Divide9/2, Divide7/1, Square1/1
  Square1/1 -> Add3/2
  Square/1 -> Add3/1
  Divide6/1 -> Add9/1
  Divide9/1 -> Add9/2
  Add9/1 -> Divide/1
  Divide7/1 -> Add8/1
  Demux/1 -> [Vd], Divide6/2, Square/1, Divide14/2
  Pref/1 -> Divide6/1, Divide7/2
  id*3/1 -> Divide15/1
  Divide15/1 -> Saturation4/1
  Qref/1 -> Divide14/1, Divide9/1
  Divide14/1 -> Add8/2
  Saturation4/1 -> Divide1/1, Divide/2
  Add3/1 -> Divide15/2
  Vdq/1 -> Demux/1
  Divide/1 -> Mux2/1
  Divide1/1 -> Mux2/2
  Add8/1 -> Divide1/2
  Mux2/1 -> IdqRef/1

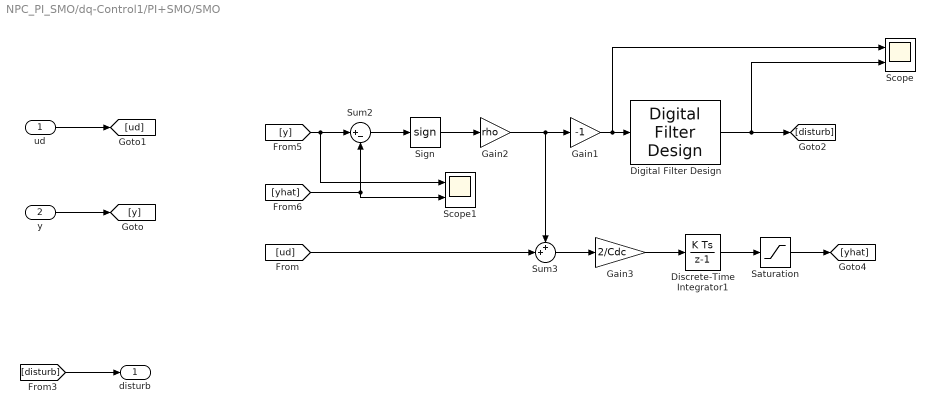
== system NPC_PI_SMO/dq-Control1/PI+SMO/SMO ==
  ud : Inport
  y : Inport  Port=2
  Digital Filter Design : dsparch4/Digital Filter Design  mwdsp_browser_bugfix_var=off
  Discrete-Time Integrator1 : DiscreteIntegrator  SampleTime=-1  ICPrevOutput=DiscIntNeverNeededParam  ICPrevScaledInput=DiscIntNeverNeededParam
  Gain1 : Gain  Gain=-1
  Gain2 : Gain  Gain=rho
  Gain3 : Gain  Gain=2/Cdc
  Saturation : Saturate  UpperLimit=5e6
  Scope : Scope  NumInputPorts=2
  Scope1 : Scope  NumInputPorts=2
  Sign : Signum
  Sum2 : Sum  Inputs=|+-
  Sum3 : Sum  Inputs=++|
  disturb : Outport
  wires:
  Discrete-Time Integrator1/1 -> Saturation/1
  Gain3/1 -> Discrete-Time Integrator1/1
  Sum3/1 -> Gain3/1
  Gain2/1 -> Gain1/1, Sum3/1
  Sum2/1 -> Sign/1
  [y] -> Scope1/1, Sum2/1
  [ud] -> Sum3/2
  [disturb] -> disturb/1
  ud/1 -> [ud]
  y/1 -> [y]
  Saturation/1 -> [yhat]
  Sign/1 -> Gain2/1
  Digital Filter Design/1 -> [disturb], Scope/2
  Gain1/1 -> Scope/1, Digital Filter Design/1
  [yhat] -> Sum2/2, Scope1/2
